simulink model "request_buffer_test"  (R2021b)
settings: Solver=VariableStepAuto  StartTime=0.0  StopTime=stop_time  RelTol=1e-3
values from neighbouring files (symbols this model uses):
  input_bus = make_input(     empty(3),      req_ut(1, 1, 1, 1, 1),      empty(),      req_uc(2, 2, 1, 20, 1),      empty(),      req(3, 2,  2,  2, 21, 1),      empty(),      req(4, 2, 63, 63, 22, 1),      empty(),      req_send(5, 2, 64, 64, 23, 1),      empty(),      req(6, 2,  1,  1, 24, 1),      empty(),      req(7, 2,  3,  2, 25, 1),      empty(2),      req_cancel(4),      req_cancel(cancel_id_error),      ...(+56 chars)    [request_buffer_testground.m]
libraries: dspsrcs4 x22
settings Model: Creator=torha  LastModifiedBy=torha
settings SolverCC: AlgebraicLoopSolver=TrustRegion
settings DebuggingCC: SFMachineParentedDataDiag=warning

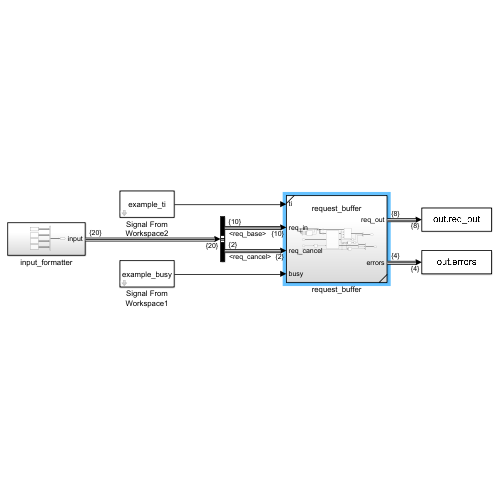
[thumbnail: Simulink's stored preview of the top-level diagram]
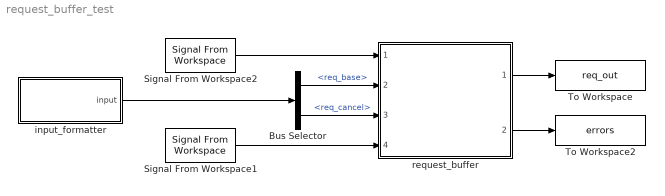
== system request_buffer_test ==
  Bus Selector : BusSelector  OutputSignals=req_base,req_cancel
  Signal From Workspace1 : dspsrcs4/Signal From Workspace  X=example_busy  Ts=1  nsamps=1  OutputAfterFinalValue=Setting to zero  ignoreOrWarnInputAndFrameLengths=off  OutputFrames=off
  Signal From Workspace2 : dspsrcs4/Signal From Workspace  X=example_ti  Ts=1  nsamps=1  OutputAfterFinalValue=Setting to zero  ignoreOrWarnInputAndFrameLengths=off  OutputFrames=off
  To Workspace : ToWorkspace  VariableName=req_out  SaveFormat=Timeseries  SampleTime=-1
      settings: Save2DSignal=2-D array (concatenate along first dimension)
  To Workspace2 : ToWorkspace  VariableName=errors  SaveFormat=Timeseries  SampleTime=-1
      settings: Save2DSignal=2-D array (concatenate along first dimension)
  input_formatter : Subsystem
  request_buffer : Subsystem  ReferencedSubsystem=request_buffer
  wires:
  Signal From Workspace1/1 -> request_buffer/4
  request_buffer/1 -> To Workspace/1
  request_buffer/2 -> To Workspace2/1
  Signal From Workspace2/1 -> request_buffer/1
  input_formatter/1(input) -> Bus Selector/1
  Bus Selector/1 -> request_buffer/2  "<req_base>"
  Bus Selector/2 -> request_buffer/3  "<req_cancel>"

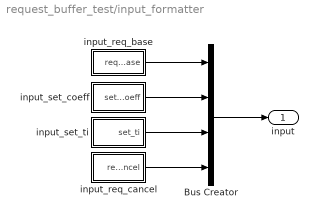
== system request_buffer_test/input_formatter ==
  Bus Creator : BusCreator  Inputs=4
  input_req_base : Subsystem
  input_req_cancel : Subsystem
  input_set_coeff : Subsystem
  input_set_ti : Subsystem
  input : Outport
  wires:
  input_req_cancel/1(req_cancel) -> Bus Creator/4
  input_set_ti/1(set_ti) -> Bus Creator/3
  input_set_coeff/1(set_coeff) -> Bus Creator/2
  input_req_base/1(req_base) -> Bus Creator/1
  Bus Creator/1 -> input/1

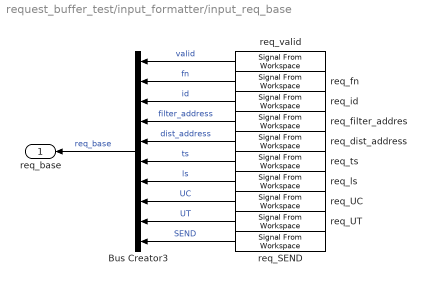
== system request_buffer_test/input_formatter/input_req_base ==
  Bus Creator3 : BusCreator  Inputs=10
  req_SEND : dspsrcs4/Signal From Workspace  X=[horzcat([input_bus.req_base]).SEND].'  Ts=1  nsamps=1  OutputAfterFinalValue=Setting to zero  ignoreOrWarnInputAndFrameLengths=off  OutputFrames=off
  req_UC : dspsrcs4/Signal From Workspace  X=[horzcat([input_bus.req_base]).UC].'  Ts=1  nsamps=1  OutputAfterFinalValue=Setting to zero  ignoreOrWarnInputAndFrameLengths=off  OutputFrames=off
  req_UT : dspsrcs4/Signal From Workspace  X=[horzcat([input_bus.req_base]).UT].'  Ts=1  nsamps=1  OutputAfterFinalValue=Setting to zero  ignoreOrWarnInputAndFrameLengths=off  OutputFrames=off
  req_dist_address : dspsrcs4/Signal From Workspace  X=[horzcat([input_bus.req_base]).dist_address].'  Ts=1  nsamps=1  OutputAfterFinalValue=Setting to zero  ignoreOrWarnInputAndFrameLengths=off  OutputFrames=off
  req_filter_addres : dspsrcs4/Signal From Workspace  X=[horzcat([input_bus.req_base]).filter_address].'  Ts=1  nsamps=1  OutputAfterFinalValue=Setting to zero  ignoreOrWarnInputAndFrameLengths=off  OutputFrames=off
  req_fn : dspsrcs4/Signal From Workspace  X=[horzcat([input_bus.req_base]).fn].'  Ts=1  nsamps=1  OutputAfterFinalValue=Setting to zero  ignoreOrWarnInputAndFrameLengths=off  OutputFrames=off
  req_id : dspsrcs4/Signal From Workspace  X=[horzcat([input_bus.req_base]).id].'  Ts=1  nsamps=1  OutputAfterFinalValue=Setting to zero  ignoreOrWarnInputAndFrameLengths=off  OutputFrames=off
  req_ls : dspsrcs4/Signal From Workspace  X=[horzcat([input_bus.req_base]).ls].'  Ts=1  nsamps=1  OutputAfterFinalValue=Setting to zero  ignoreOrWarnInputAndFrameLengths=off  OutputFrames=off
  req_ts : dspsrcs4/Signal From Workspace  X=[horzcat([input_bus.req_base]).ts].'  Ts=1  nsamps=1  OutputAfterFinalValue=Setting to zero  ignoreOrWarnInputAndFrameLengths=off  OutputFrames=off
  req_valid : dspsrcs4/Signal From Workspace  X=[horzcat([input_bus.req_base]).valid].'  Ts=1  nsamps=1  OutputAfterFinalValue=Setting to zero  ignoreOrWarnInputAndFrameLengths=off  OutputFrames=off
  req_base : Outport
  wires:
  req_UC/1 -> Bus Creator3/8  "UC"
  req_filter_addres/1 -> Bus Creator3/4  "filter_address"
  req_dist_address/1 -> Bus Creator3/5  "dist_address"
  req_fn/1 -> Bus Creator3/2  "fn"
  req_UT/1 -> Bus Creator3/9  "UT"
  req_SEND/1 -> Bus Creator3/10  "SEND"
  req_valid/1 -> Bus Creator3/1  "valid"
  req_ls/1 -> Bus Creator3/7  "ls"
  req_id/1 -> Bus Creator3/3  "id"
  req_ts/1 -> Bus Creator3/6  "ts"
  Bus Creator3/1 -> req_base/1  "req_base"

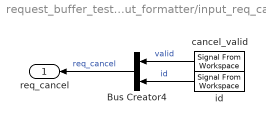
== system request_buffer_test/input_formatter/input_req_cancel ==
  Bus Creator4 : BusCreator  Inputs=2
  cancel_valid : dspsrcs4/Signal From Workspace  X=[horzcat([input_bus.req_cancel]).valid].'  Ts=1  nsamps=1  OutputAfterFinalValue=Setting to zero  ignoreOrWarnInputAndFrameLengths=off  OutputFrames=off
  id : dspsrcs4/Signal From Workspace  X=[horzcat([input_bus.req_cancel]).id].'  Ts=1  nsamps=1  OutputAfterFinalValue=Setting to zero  ignoreOrWarnInputAndFrameLengths=off  OutputFrames=off
  req_cancel : Outport
  wires:
  id/1 -> Bus Creator4/2  "id"
  cancel_valid/1 -> Bus Creator4/1  "valid"
  Bus Creator4/1 -> req_cancel/1  "req_cancel"

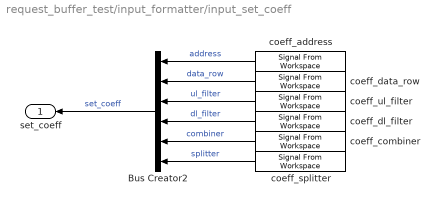
== system request_buffer_test/input_formatter/input_set_coeff ==
  Bus Creator2 : BusCreator  Inputs=6
  coeff_address : dspsrcs4/Signal From Workspace  X=[horzcat([input_bus.set_coeff]).address].'  Ts=1  nsamps=1  OutputAfterFinalValue=Setting to zero  ignoreOrWarnInputAndFrameLengths=off  OutputFrames=off
  coeff_combiner : dspsrcs4/Signal From Workspace  X=[horzcat([input_bus.set_coeff]).combiner].'  Ts=1  nsamps=1  OutputAfterFinalValue=Setting to zero  ignoreOrWarnInputAndFrameLengths=off  OutputFrames=off
  coeff_data_row : dspsrcs4/Signal From Workspace  X=[horzcat([input_bus.set_coeff]).data_row].'  Ts=1  nsamps=1  OutputAfterFinalValue=Setting to zero  ignoreOrWarnInputAndFrameLengths=off  OutputFrames=off
  coeff_dl_filter : dspsrcs4/Signal From Workspace  X=[horzcat([input_bus.set_coeff]).dl_filter].'  Ts=1  nsamps=1  OutputAfterFinalValue=Setting to zero  ignoreOrWarnInputAndFrameLengths=off  OutputFrames=off
  coeff_splitter : dspsrcs4/Signal From Workspace  X=[horzcat([input_bus.set_coeff]).splitter].'  Ts=1  nsamps=1  OutputAfterFinalValue=Setting to zero  ignoreOrWarnInputAndFrameLengths=off  OutputFrames=off
  coeff_ul_filter : dspsrcs4/Signal From Workspace  X=[horzcat([input_bus.set_coeff]).ul_filter].'  Ts=1  nsamps=1  OutputAfterFinalValue=Setting to zero  ignoreOrWarnInputAndFrameLengths=off  OutputFrames=off
  set_coeff : Outport
  wires:
  coeff_ul_filter/1 -> Bus Creator2/3  "ul_filter"
  coeff_dl_filter/1 -> Bus Creator2/4  "dl_filter"
  coeff_address/1 -> Bus Creator2/1  "address"
  coeff_splitter/1 -> Bus Creator2/6  "splitter"
  coeff_data_row/1 -> Bus Creator2/2  "data_row"
  coeff_combiner/1 -> Bus Creator2/5  "combiner"
  Bus Creator2/1 -> set_coeff/1  "set_coeff"

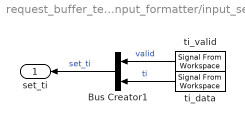
== system request_buffer_test/input_formatter/input_set_ti ==
  Bus Creator1 : BusCreator  Inputs=2
  ti_data : dspsrcs4/Signal From Workspace  X=[horzcat([input_bus.set_ti]).ti].'  Ts=1  nsamps=1  OutputAfterFinalValue=Setting to zero  ignoreOrWarnInputAndFrameLengths=off  OutputFrames=off
  ti_valid : dspsrcs4/Signal From Workspace  X=[horzcat([input_bus.set_ti]).valid].'  Ts=1  nsamps=1  OutputAfterFinalValue=Setting to zero  ignoreOrWarnInputAndFrameLengths=off  OutputFrames=off
  set_ti : Outport
  wires:
  ti_valid/1 -> Bus Creator1/1  "valid"
  ti_data/1 -> Bus Creator1/2  "ti"
  Bus Creator1/1 -> set_ti/1  "set_ti"
